simulink model "lcc"  (R2025a)
settings: Solver=VariableStepAuto  StartTime=0.0  StopTime=10.0  RelTol=1e-3
settings Model: Creator=matthewkeller  LastModifiedBy=matthewkeller

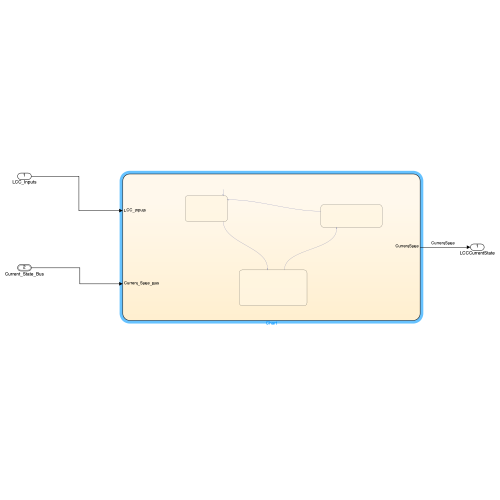
[thumbnail: Simulink's stored preview of the top-level diagram]
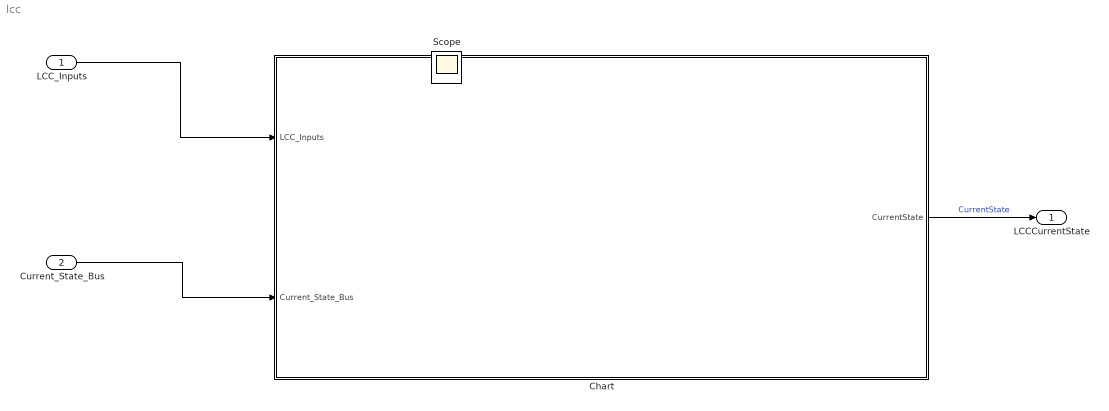
== system lcc ==
  LCC_Inputs : Inport
  Current_State_Bus : Inport  Port=2  OutDataTypeStr=Bus: CurrentStateBus
  Chart : Stateflow chart  TreatAsAtomicUnit=on
  LCCCurrentState : Outport
  Scope : Scope
      settings: ActiveDisplayYMinimum=-1  ActiveDisplayYMaximum=1
  wires:
  Chart/1(CurrentState) -> LCCCurrentState/1  "CurrentState"
  LCC_Inputs/1 -> Chart/1(LCC_Inputs)
  Current_State_Bus/1 -> Chart/2(Current_State_Bus)

== stateflow chart lcc/Chart ==
  settings: executeAtInitialization=1
  state LCC_Deactivated
    entry:
    CurrentState = 0;
  state LCC_Active
    entry:
    CurrentState = 2;
  state LCC_Standby
    entry:
    CurrentState = 1;
  (default) -> LCC_Deactivated
  LCC_Active -> LCC_Deactivated : [LCC_Inputs.Cancel_LCC_Pressed]
  LCC_Deactivated -> LCC_Standby : [LCC_Inputs.Lane_Change_Centred && LCC_Inputs.Speed_GT_35_MPH && LCC_Inputs.Lateral_Switch_ON && Current_State_Bus.APStatus == 0]
  LCC_Standby -> LCC_Active : [LCC_Inputs.Activate_LCC_Pressed]
  data: LCC_Inputs input Bus: LCCStatusBus; CurrentState output int8; Current_State_Bus input Bus: CurrentStateBus
